simulink model "main"  (R2022a)
settings: Solver=FixedStepDiscrete  StartTime=0.0  StopTime=Inf  FixedStep=(50e-6)-(sim_en*4.995e-5)  RelTol=1e-3  EnableMultiTasking=on
model workspace (MAT data in the model file):
  Param : Simulink.Parameter (value not decoded)
  ac_ok : Simulink.Signal (value not decoded)
  ac_ok_120 : Simulink.Signal (value not decoded)
  bulk_voltage : Simulink.Signal (value not decoded)
  burstduty_integ_max : Simulink.Signal (value not decoded)
  burstduty_integ_min : Simulink.Signal (value not decoded)
  burstduty_ki : Simulink.Signal (value not decoded)
  burstduty_kp : Simulink.Signal (value not decoded)
  calib_ok : Simulink.Signal (value not decoded)
  can_addr1 : Simulink.Signal (value not decoded)
  can_addr2 : Simulink.Signal (value not decoded)
  can_addr3 : Simulink.Signal (value not decoded)
  can_addr4 : Simulink.Signal (value not decoded)
  can_data_rx : Simulink.Signal (value not decoded)
  can_data_tx : Simulink.Signal (value not decoded)
  can_timeout_120 : Simulink.Signal (value not decoded)
  chksum_scircv : Simulink.Signal (value not decoded)
  clllc_en_120 : Simulink.Signal (value not decoded)
  clllc_fault_120 : Simulink.Signal (value not decoded)
  clllc_ok_120 : Simulink.Signal (value not decoded)
  cmpss1h : Simulink.Signal (value not decoded)
  cmpss1l : Simulink.Signal (value not decoded)
  cmpss2h : Simulink.Signal (value not decoded)
  cmpss2l : Simulink.Signal (value not decoded)
  cmpss3h : Simulink.Signal (value not decoded)
  cmpss3l : Simulink.Signal (value not decoded)
  cmpss4h : Simulink.Signal (value not decoded)
  cmpss4l : Simulink.Signal (value not decoded)
  cmpss5h : Simulink.Signal (value not decoded)
  cmpss5l : Simulink.Signal (value not decoded)
  cmpss6h : Simulink.Signal (value not decoded)
  cmpss6l : Simulink.Signal (value not decoded)
  cmpss7h : Simulink.Signal (value not decoded)
  cmpss7l : Simulink.Signal (value not decoded)
  cmpss8h : Simulink.Signal (value not decoded)
  cmpss8l : Simulink.Signal (value not decoded)
  cnt_idle : Simulink.Signal (value not decoded)
  cnt_orps : Simulink.Signal (value not decoded)
  cnt_scircv : Simulink.Signal (value not decoded)
  cnt_scixmt : Simulink.Signal (value not decoded)
  cnt_scixmt_func : Simulink.Signal (value not decoded)
  cnt_temp_mux : Simulink.Signal (value not decoded)
  cnt_vdroop : Simulink.Signal (value not decoded)
  config_ok : Simulink.Signal (value not decoded)
  control_en : Simulink.Signal (value not decoded)
  cp_ready_120 : Simulink.Signal (value not decoded)
  d2d_en : Simulink.Signal (value not decoded)
  dchg_off : Simulink.Signal (value not decoded)
  debug_dacb : Simulink.Signal (value not decoded)
  debug_dacc : Simulink.Signal (value not decoded)
  debug_msg1 : Simulink.Signal (value not decoded)
  debug_msg2 : Simulink.Signal (value not decoded)
  debug_msg3 : Simulink.Signal (value not decoded)
  debug_msg4 : Simulink.Signal (value not decoded)
  debug_msg5 : Simulink.Signal (value not decoded)
  debug_msg6 : Simulink.Signal (value not decoded)
  dir_v2g : Simulink.Signal (value not decoded)
  eoss_llc1 : Simulink.Signal (value not decoded)
  eoss_llc2 : Simulink.Signal (value not decoded)
  eoss_orps : Simulink.Signal (value not decoded)
  fault_ocp : Simulink.Signal (value not decoded)
  fault_otp : Simulink.Signal (value not decoded)
  fault_ovp : Simulink.Signal (value not decoded)
  fut_en : Simulink.Signal (value not decoded)
  fwd_en_120 : Simulink.Signal (value not decoded)
  gain_llc1_sec_idc : Simulink.Signal (value not decoded)
  gain_llc1_temp_sr : Simulink.Signal (value not decoded)
  gain_llc2_sec_idc : Simulink.Signal (value not decoded)
  gain_vbat : Simulink.Signal (value not decoded)
  gain_vbulk : Simulink.Signal (value not decoded)
  gain_vout : Simulink.Signal (value not decoded)
  input_current_phasea : Simulink.Signal (value not decoded)
  input_current_phaseb : Simulink.Signal (value not decoded)
  input_current_phasec : Simulink.Signal (value not decoded)
  input_freq : Simulink.Signal (value not decoded)
  input_power : Simulink.Signal (value not decoded)
  input_voltage_phasea : Simulink.Signal (value not decoded)
  input_voltage_phaseb : Simulink.Signal (value not decoded)
  input_voltage_phasec : Simulink.Signal (value not decoded)
  ishare_arbiter : Simulink.Signal (value not decoded)
  ishare_thresh : Simulink.Signal (value not decoded)
  led_g : Simulink.Signal (value not decoded)
  led_r : Simulink.Signal (value not decoded)
  led_y : Simulink.Signal (value not decoded)
  llc1_burst_integ : Simulink.Signal (value not decoded)
  llc1_burstduty_buffer : Simulink.Signal (value not decoded)
  llc1_pfm_error : Simulink.Signal (value not decoded)
  llc1_pfm_integ : Simulink.Signal (value not decoded)
  llc1_pfm_prop : Simulink.Signal (value not decoded)
  llc1_pri_idc : Simulink.Signal (value not decoded)
  llc1_ps_buffer : Simulink.Signal (value not decoded)
  llc1_pspwm_error : Simulink.Signal (value not decoded)
  llc1_pspwm_integ : Simulink.Signal (value not decoded)
  llc1_pspwm_prop : Simulink.Signal (value not decoded)
  llc1_sec_idc : Simulink.Signal (value not decoded)
  llc1_temp_sr : Simulink.Signal (value not decoded)
  llc1_ts_tbctr_buffer : Simulink.Signal (value not decoded)
  llc2_burst_integ : Simulink.Signal (value not decoded)
  llc2_burstduty_buffer : Simulink.Signal (value not decoded)
  llc2_en : Simulink.Signal (value not decoded)
  llc2_en_buffer : Simulink.Signal (value not decoded)
  llc2_pfm_error : Simulink.Signal (value not decoded)
  llc2_pfm_integ : Simulink.Signal (value not decoded)
  llc2_pfm_prop : Simulink.Signal (value not decoded)
  llc2_pri_idc : Simulink.Signal (value not decoded)
  llc2_ps_buffer : Simulink.Signal (value not decoded)
  llc2_pspwm_error : Simulink.Signal (value not decoded)
  llc2_pspwm_integ : Simulink.Signal (value not decoded)
  llc2_pspwm_prop : Simulink.Signal (value not decoded)
  llc2_sec_idc : Simulink.Signal (value not decoded)
  llc2_temp_sr : Simulink.Signal (value not decoded)
  llc2_ts_tbctr_buffer : Simulink.Signal (value not decoded)
  loop_adcint : Simulink.Signal (value not decoded)
  loop_control : Simulink.Signal (value not decoded)
  loop_idle : Simulink.Signal (value not decoded)
  mid_bulk_voltage : Simulink.Signal (value not decoded)
  mode_120 : Simulink.Signal (value not decoded)
  mode_cc_cv : Simulink.Signal (value not decoded)
  myParam : mpt.Parameter (value not decoded)
  obc_ok_120 : Simulink.Signal (value not decoded)
  offset_llc1_sec_idc : Simulink.Signal (value not decoded)
  offset_llc1_temp_sr : Simulink.Signal (value not decoded)
  offset_llc2_sec_idc : Simulink.Signal (value not decoded)
  offset_vbat : Simulink.Signal (value not decoded)
  offset_vbulk : Simulink.Signal (value not decoded)
  offset_vout : Simulink.Signal (value not decoded)
  openloop_en : Simulink.Signal (value not decoded)
  openloop_fault_en : Simulink.Signal (value not decoded)
  ot_fault_120 : Simulink.Signal (value not decoded)
  pfc_en : Simulink.Signal (value not decoded)
  pfc_en_120 : Simulink.Signal (value not decoded)
  pfc_fw_revision : Simulink.Signal (value not decoded)
  pfc_fw_revision_bootloader : Simulink.Signal (value not decoded)
  pfc_fw_revision_debug : Simulink.Signal (value not decoded)
  pfc_ok : Simulink.Signal (value not decoded)
  pfc_ok_120 : Simulink.Signal (value not decoded)
  pfm_a0 : Simulink.Signal (value not decoded)
  pfm_a1 : Simulink.Signal (value not decoded)
  pfm_integ_max : Simulink.Signal (value not decoded)
  pfm_integ_min : Simulink.Signal (value not decoded)
  pfm_ki : Simulink.Signal (value not decoded)
  pfm_kp : Simulink.Signal (value not decoded)
  pri_fut_en : Simulink.Signal (value not decoded)
  pri_fut_en_buffer : Simulink.Signal (value not decoded)
  pri_halfbridge_en : Simulink.Signal (value not decoded)
  pri_halfbridge_en_buffer : Simulink.Signal (value not decoded)
  pspwm_integ_max : Simulink.Signal (value not decoded)
  pspwm_integ_min : Simulink.Signal (value not decoded)
  pspwm_ki : Simulink.Signal (value not decoded)
  pspwm_kp : Simulink.Signal (value not decoded)
  ref_idclink_max : Simulink.Signal (value not decoded)
  ref_iout : Simulink.Signal (value not decoded)
  ref_iout_calib : Simulink.Signal (value not decoded)
  ref_iout_llc1 : Simulink.Signal (value not decoded)
  ref_iout_llc1_calib : Simulink.Signal (value not decoded)
  ref_iout_llc2 : Simulink.Signal (value not decoded)
  ref_iout_llc2_calib : Simulink.Signal (value not decoded)
  ref_pout : Simulink.Signal (value not decoded)
  ref_ss_llc1 : Simulink.Signal (value not decoded)
  ref_ss_llc2 : Simulink.Signal (value not decoded)
  ref_ss_orps : Simulink.Signal (value not decoded)
  ref_vbat : Simulink.Signal (value not decoded)
  ref_vbat_calib : Simulink.Signal (value not decoded)
  ref_vbulk : Simulink.Signal (value not decoded)
  ref_vbulk_calib : Simulink.Signal (value not decoded)
  ref_vbulk_llc1_calib : Simulink.Signal (value not decoded)
  ref_vbulk_llc2_calib : Simulink.Signal (value not decoded)
  ref_vout : Simulink.Signal (value not decoded)
  ref_vout_calib : Simulink.Signal (value not decoded)
  relay_en : Simulink.Signal (value not decoded)
  reset_flag : Simulink.Signal (value not decoded)
  rev_en_120 : Simulink.Signal (value not decoded)
  runtime_control : Simulink.Signal (value not decoded)
  runtime_idle : Simulink.Signal (value not decoded)
  scircv_buffer : Simulink.Signal (value not decoded)
  scircv_buffer_tmp : Simulink.Signal (value not decoded)
  scircv_buffer_tmp_idx0 : Simulink.Signal (value not decoded)
  scircv_chksum : Simulink.Signal (value not decoded)
  scircv_chksum_ok : Simulink.Signal (value not decoded)
  scircv_parse_ok : Simulink.Signal (value not decoded)
  scixmt_buffer : Simulink.Signal (value not decoded)
  scixmt_chksum : Simulink.Signal (value not decoded)
  scixmt_func : Simulink.Signal (value not decoded)
  scixmt_word0_lsb : Simulink.Signal (value not decoded)
  scixmt_word0_msb : Simulink.Signal (value not decoded)
  scixmt_word1_lsb : Simulink.Signal (value not decoded)
  scixmt_word1_msb : Simulink.Signal (value not decoded)
  scixmt_word2_lsb : Simulink.Signal (value not decoded)
  scixmt_word2_msb : Simulink.Signal (value not decoded)
  scixmt_wr : Simulink.Signal (value not decoded)
  ss_step : Simulink.Signal (value not decoded)
  state_calib : Simulink.Signal (value not decoded)
  state_control : Simulink.Signal (value not decoded)
  state_hkeep : Simulink.Signal (value not decoded)
  status_cmpss : Simulink.Signal (value not decoded)
  status_control : Simulink.Signal (value not decoded)
  status_digin : Simulink.Signal (value not decoded)
  status_digout : Simulink.Signal (value not decoded)
  status_fault : Simulink.Signal (value not decoded)
  status_input : Simulink.Signal (value not decoded)
  status_pfc : Simulink.Signal (value not decoded)
  temp_inlet : Simulink.Signal (value not decoded)
  temp_llc1_fet_hs : Simulink.Signal (value not decoded)
  temp_llc2_fet_hs : Simulink.Signal (value not decoded)
  temp_mux : Simulink.Signal (value not decoded)
  temp_mux_s0 : Simulink.Signal (value not decoded)
  temp_mux_s1 : Simulink.Signal (value not decoded)
  temp_mux_s2 : Simulink.Signal (value not decoded)
  temp_outlet : Simulink.Signal (value not decoded)
  temp_pfc_fet_hsa : Simulink.Signal (value not decoded)
  temp_pfc_fet_hsb : Simulink.Signal (value not decoded)
  temp_pfc_fet_hsc : Simulink.Signal (value not decoded)
  temp_pfc_fet_lsa : Simulink.Signal (value not decoded)
  temp_pfc_fet_lsb : Simulink.Signal (value not decoded)
  temp_pfc_fet_lsc : Simulink.Signal (value not decoded)
  test_mode : Simulink.Signal (value not decoded)
  tfcv_cc : Simulink.Signal (value not decoded)
  tfcv_cc_llc2 : Simulink.Signal (value not decoded)
  tfcv_cv : Simulink.Signal (value not decoded)
  tfcv_sr_en : Simulink.Signal (value not decoded)
  tfv_assert_llc1_pri_idc : Simulink.Signal (value not decoded)
  tfv_assert_llc1_sec_idc : Simulink.Signal (value not decoded)
  tfv_assert_llc1_temp_sr : Simulink.Signal (value not decoded)
  tfv_assert_llc2_pri_idc : Simulink.Signal (value not decoded)
  tfv_assert_llc2_sec_idc : Simulink.Signal (value not decoded)
  tfv_assert_llc2_temp_sr : Simulink.Signal (value not decoded)
  tfv_assert_temp_outlet : Simulink.Signal (value not decoded)
  tfv_assert_vaux_uv : Simulink.Signal (value not decoded)
  tfv_assert_vbat : Simulink.Signal (value not decoded)
  tfv_assert_vbulk : Simulink.Signal (value not decoded)
  tfv_assert_vout : Simulink.Signal (value not decoded)
  tfv_cnt_tz : Simulink.Signal (value not decoded)
  tfv_deassert_llc1_pri_idc : Simulink.Signal (value not decoded)
  tfv_deassert_llc1_sec_idc : Simulink.Signal (value not decoded)
  tfv_deassert_llc1_temp_sr : Simulink.Signal (value not decoded)
  tfv_deassert_llc2_pri_idc : Simulink.Signal (value not decoded)
  tfv_deassert_llc2_sec_idc : Simulink.Signal (value not decoded)
  tfv_deassert_llc2_temp_sr : Simulink.Signal (value not decoded)
  tfv_deassert_temp_outlet : Simulink.Signal (value not decoded)
  tfv_deassert_vaux_uv : Simulink.Signal (value not decoded)
  tfv_deassert_vbat : Simulink.Signal (value not decoded)
  tfv_deassert_vbulk : Simulink.Signal (value not decoded)
  tfv_deassert_vout : Simulink.Signal (value not decoded)
  tfv_llc1_pri_idc : Simulink.Signal (value not decoded)
  tfv_llc1_sec_idc : Simulink.Signal (value not decoded)
  tfv_llc1_temp_sr : Simulink.Signal (value not decoded)
  tfv_llc2_pri_idc : Simulink.Signal (value not decoded)
  tfv_llc2_sec_idc : Simulink.Signal (value not decoded)
  tfv_llc2_temp_sr : Simulink.Signal (value not decoded)
  tfv_temp_outlet : Simulink.Signal (value not decoded)
  tfv_vaux_uv : Simulink.Signal (value not decoded)
  tfv_vbat : Simulink.Signal (value not decoded)
  tfv_vbulk : Simulink.Signal (value not decoded)
  tfv_vout : Simulink.Signal (value not decoded)
  timer_1ms : Simulink.Signal (value not decoded)
  tz : Simulink.Signal (value not decoded)
  valve_en : Simulink.Signal (value not decoded)
  vaux : Simulink.Signal (value not decoded)
  vbat : Simulink.Signal (value not decoded)
  vbulk : Simulink.Signal (value not decoded)
  vout : Simulink.Signal (value not decoded)
undefined symbols (not defined in the file or in its folder): CAN_O_INT, CANA_BASE, Down, GPTRIP1SEL, GPTRIP2SEL, TZ1, TZ2, Up
libraries: hdlsllib x159, simulink x94, c2802xlib x32, c2837xDlib x19, c2807xlib x16, c280xlib x13, canmsglib x8, idelinklib_common x2, c2000lib x1, c281xlib x1
(part 11 of 20)

== system main/Task_Manager/idle/idle_task/hkeep/tz ==
  note: //Code:
      | main_DWork.tz_sc = (uint16_T)(EPwm1Regs.TZOSTFLG.bit.OST1);
      | main_DWork.tz_oc = (uint16_T)(EPwm1Regs.TZOSTFLG.bit.OST2);
      | main_DWork.tz_ov = (uint16_T)(EPwm1Regs.TZOSTFLG.bit.OST3);
  note: main_DWork.tz = (uint16_T)(EPwm1Regs.TZOSTFLG.bit.OST3);
  note: main_DWork.tz = (uint16_T)(EPwm1Regs.TZCBCFLG.bit.CBC3);
  note: //Code:
      | main_DWork.tz_ov = (uint16_T)(EPwm1Regs.TZOSTFLG.bit.OST1); //X-BAR GPIO61 VBULK and VBAT OVP
      | //main_DWork.tz_ocp1 = (uint16_T)(EPwm1Regs.TZOSTFLG.bit.OST2); //X-BAR GPIO62 IOUT OCP
      | //main_DWork.tz_ocp2 = (uint16_T)(EPwm1Regs.TZOSTFLG.bit.OST3); //X-BAR GPIO63 ITANK OCP
  function : TriggerPort  TriggerType=function-call  VariantControl=Variant
  System Outputs : Subsystem  Commented=on  mask(System Outputs){ShowInLibBrowser=0}
      mask prompts: ShowInLibBrowser "Simulink:masks:CustCodeMaskParam1_MP"
      settings: CopyFcn=cccopyfcn(gcb)  OpenFcn=ccopenfcn('System Outputs Function')
      mask Help: eval('feval(''rtwprivate'',''rtwhelpview'',''rtw_sys_outputs_block'')');
      mask Display: disp('System\nOutputs');
  System Outputs1 : Subsystem  Commented=on  mask(System Outputs){ShowInLibBrowser=0}
      mask prompts: ShowInLibBrowser "Simulink:masks:CustCodeMaskParam1_MP"
      settings: CopyFcn=cccopyfcn(gcb)  OpenFcn=ccopenfcn('System Outputs Function')
      mask Help: eval('feval(''rtwprivate'',''rtwhelpview'',''rtw_sys_outputs_block'')');
      mask Display: disp('System\nOutputs');
  System Outputs2 : Subsystem  Commented=on  mask(System Outputs){ShowInLibBrowser=0}
      mask prompts: ShowInLibBrowser "Simulink:masks:CustCodeMaskParam1_MP"
      settings: CopyFcn=cccopyfcn(gcb)  OpenFcn=ccopenfcn('System Outputs Function')
      mask Help: eval('feval(''rtwprivate'',''rtwhelpview'',''rtw_sys_outputs_block'')');
      mask Display: disp('System\nOutputs');
  System Outputs3 : Subsystem  Commented=on  mask(System Outputs){ShowInLibBrowser=0}
      mask prompts: ShowInLibBrowser "Simulink:masks:CustCodeMaskParam1_MP"
      settings: CopyFcn=cccopyfcn(gcb)  OpenFcn=ccopenfcn('System Outputs Function')
      mask Help: eval('feval(''rtwprivate'',''rtwhelpview'',''rtw_sys_outputs_block'')');
      mask Display: disp('System\nOutputs');
  System Outputs4 : Subsystem  mask(System Outputs){ShowInLibBrowser=0}
      mask prompts: ShowInLibBrowser "Simulink:masks:CustCodeMaskParam1_MP"
      settings: CopyFcn=cccopyfcn(gcb)  OpenFcn=ccopenfcn('System Outputs Function')
      mask Help: eval('feval(''rtwprivate'',''rtwhelpview'',''rtw_sys_outputs_block'')');
      mask Display: disp('System\nOutputs');

== system main/Task_Manager/idle/idle_task/status/init ==
  sim_digin : Inport
  function : TriggerPort  TriggerType=function-call  VariantControl=Variant
  digin/digout_variant_subsystem : Subsystem  Variant=on
  sim_digout : Outport
  wires:
  sim_digin/1 -> digin/digout_variant_subsystem/1(sim_digin)
  digin/digout_variant_subsystem/1(sim_digout) -> sim_digout/1

== system main/Task_Manager/idle/idle_task/status/status_control ==
  function : TriggerPort  TriggerType=function-call  VariantControl=Variant
  Add : Sum  Inputs=+++++++++++
  Bit Shift1 : hdlsllib/Logic and Bit Operations/Bit Shift  mode=Shift Left Logical  N=1
  Bit Shift10 : hdlsllib/Logic and Bit Operations/Bit Shift  mode=Shift Left Logical  N=10
  Bit Shift2 : hdlsllib/Logic and Bit Operations/Bit Shift  mode=Shift Left Logical  N=2
  Bit Shift3 : hdlsllib/Logic and Bit Operations/Bit Shift  mode=Shift Left Logical  N=3
  Bit Shift4 : hdlsllib/Logic and Bit Operations/Bit Shift  mode=Shift Left Logical  N=5
  Bit Shift5 : hdlsllib/Logic and Bit Operations/Bit Shift  mode=Shift Left Logical  N=6
  Bit Shift6 : hdlsllib/Logic and Bit Operations/Bit Shift  mode=Shift Left Logical  N=4
  Bit Shift7 : hdlsllib/Logic and Bit Operations/Bit Shift  mode=Shift Left Logical  N=7
  Bit Shift8 : hdlsllib/Logic and Bit Operations/Bit Shift  mode=Shift Left Logical  N=8
  Bit Shift9 : hdlsllib/Logic and Bit Operations/Bit Shift  mode=Shift Left Logical  N=9
  Data Store Read1 : DataStoreRead  DataStoreName=eoss_llc2  IndexOptions=Index vector (dialog)  Indices=1  OutputSizes=1
  Data Store Read10 : DataStoreRead  DataStoreName=dir_v2g  IndexOptions=Index vector (dialog)  Indices=1  OutputSizes=1
  Data Store Read11 : DataStoreRead  DataStoreName=eoss_llc1  IndexOptions=Index vector (dialog)  Indices=1  OutputSizes=1
  Data Store Read12 : DataStoreRead  DataStoreName=calib_ok  IndexOptions=Index vector (dialog)  Indices=1  OutputSizes=1
  Data Store Read13 : DataStoreRead  DataStoreName=openloop_en  IndexOptions=Index vector (dialog)  Indices=1  OutputSizes=1
  Data Store Read2 : DataStoreRead  DataStoreName=llc2_en  IndexOptions=Index vector (dialog)  Indices=1  OutputSizes=1
  Data Store Read3 : DataStoreRead  DataStoreName=pri_halfbridge_en  IndexOptions=Index vector (dialog)  Indices=1  OutputSizes=1
  Data Store Read4 : DataStoreRead  DataStoreName=config_ok  IndexOptions=Index vector (dialog)  Indices=1  OutputSizes=1
  Data Store Read5 : DataStoreRead  DataStoreName=openloop_fault_en  IndexOptions=Index vector (dialog)  Indices=1  OutputSizes=1
  Data Store Read6 : DataStoreRead  DataStoreName=control_en  IndexOptions=Index vector (dialog)  Indices=1  OutputSizes=1
  Data Store Read7 : DataStoreRead  DataStoreName=fut_en  IndexOptions=Index vector (dialog)  Indices=1  OutputSizes=1
  Data Store Write7 : DataStoreWrite  DataStoreName=status_control  IndexOptions=Index vector (dialog)  Indices=1  OutputSizes=1
  Data Type Conversion{,1..10} (11 alike) : DataTypeConversion  OutDataTypeStr=uint16  SaturateOnIntegerOverflow=off  RndMeth=Floor
  wires:
  Add/1 -> Data Store Write7/1
  Data Store Read10/1 -> Data Type Conversion1/1
  Bit Shift2/1 -> Add/3
  Data Store Read6/1 -> Data Type Conversion/1
  Bit Shift3/1 -> Add/4
  Bit Shift1/1 -> Add/2
  Bit Shift6/1 -> Add/5
  Data Type Conversion1/1 -> Bit Shift1/1
  Data Type Conversion2/1 -> Bit Shift2/1
  Data Type Conversion3/1 -> Bit Shift3/1
  Data Type Conversion4/1 -> Bit Shift6/1
  Bit Shift4/1 -> Add/6
  Data Store Read12/1 -> Data Type Conversion2/1
  Data Type Conversion5/1 -> Bit Shift4/1
  Data Type Conversion6/1 -> Bit Shift5/1
  Data Type Conversion7/1 -> Bit Shift7/1
  Data Type Conversion8/1 -> Bit Shift8/1
  Data Type Conversion9/1 -> Bit Shift9/1
  Bit Shift9/1 -> Add/10
  Bit Shift5/1 -> Add/7
  Bit Shift7/1 -> Add/8
  Bit Shift8/1 -> Add/9
  Data Type Conversion/1 -> Add/1
  Data Type Conversion10/1 -> Bit Shift10/1
  Bit Shift10/1 -> Add/11
  Data Store Read3/1 -> Data Type Conversion10/1
  Data Store Read2/1 -> Data Type Conversion9/1
  Data Store Read5/1 -> Data Type Conversion8/1
  Data Store Read13/1 -> Data Type Conversion7/1
  Data Store Read7/1 -> Data Type Conversion6/1
  Data Store Read1/1 -> Data Type Conversion5/1
  Data Store Read11/1 -> Data Type Conversion4/1
  Data Store Read4/1 -> Data Type Conversion3/1

== system main/Task_Manager/idle/idle_task/status/status_digin ==
  function : TriggerPort  TriggerType=function-call  VariantControl=Variant
  Add : Sum  Inputs=+++++++
  Bit Shift1 : hdlsllib/Logic and Bit Operations/Bit Shift  mode=Shift Left Logical  N=1
  Bit Shift2 : hdlsllib/Logic and Bit Operations/Bit Shift  mode=Shift Left Logical  N=2
  Bit Shift3 : hdlsllib/Logic and Bit Operations/Bit Shift  mode=Shift Left Logical  N=3
  Bit Shift4 : hdlsllib/Logic and Bit Operations/Bit Shift  mode=Shift Left Logical  N=5
  Bit Shift5 : hdlsllib/Logic and Bit Operations/Bit Shift  mode=Shift Left Logical  N=6
  Bit Shift6 : hdlsllib/Logic and Bit Operations/Bit Shift  mode=Shift Left Logical  N=4
  Data Store Read : DataStoreRead  DataStoreName=can_addr1  IndexOptions=Index vector (dialog)  Indices=1  OutputSizes=1
  Data Store Read1 : DataStoreRead  DataStoreName=can_addr2  IndexOptions=Index vector (dialog)  Indices=1  OutputSizes=1
  Data Store Read2 : DataStoreRead  DataStoreName=can_addr3  IndexOptions=Index vector (dialog)  Indices=1  OutputSizes=1
  Data Store Read3 : DataStoreRead  DataStoreName=can_addr4  IndexOptions=Index vector (dialog)  Indices=1  OutputSizes=1
  Data Store Read4 : DataStoreRead  DataStoreName=pfc_ok  IndexOptions=Index vector (dialog)  Indices=1  OutputSizes=1
  Data Store Read5 : DataStoreRead  DataStoreName=ac_ok  IndexOptions=Index vector (dialog)  Indices=1  OutputSizes=1
  Data Store Read6 : DataStoreRead  DataStoreName=d2d_en  IndexOptions=Index vector (dialog)  Indices=1  OutputSizes=1
  Data Store Write : DataStoreWrite  DataStoreName=status_digin  IndexOptions=Index vector (dialog)  Indices=1  OutputSizes=1
  Data Type Conversion{,1..6} (7 alike) : DataTypeConversion  OutDataTypeStr=uint16  SaturateOnIntegerOverflow=off  RndMeth=Floor
  wires:
  Data Store Read/1 -> Data Type Conversion/1
  Data Store Read1/1 -> Data Type Conversion1/1
  Data Store Read2/1 -> Data Type Conversion2/1
  Data Store Read6/1 -> Data Type Conversion6/1
  Data Store Read5/1 -> Data Type Conversion5/1
  Data Store Read4/1 -> Data Type Conversion4/1
  Data Store Read3/1 -> Data Type Conversion3/1
  Bit Shift5/1 -> Add/7
  Bit Shift4/1 -> Add/6
  Bit Shift6/1 -> Add/5
  Bit Shift3/1 -> Add/4
  Bit Shift2/1 -> Add/3
  Bit Shift1/1 -> Add/2
  Add/1 -> Data Store Write/1
  Data Type Conversion/1 -> Add/1
  Data Type Conversion1/1 -> Bit Shift1/1
  Data Type Conversion2/1 -> Bit Shift2/1
  Data Type Conversion3/1 -> Bit Shift3/1
  Data Type Conversion4/1 -> Bit Shift6/1
  Data Type Conversion5/1 -> Bit Shift4/1
  Data Type Conversion6/1 -> Bit Shift5/1

== system main/Task_Manager/idle/idle_task/status/status_digout ==
  function : TriggerPort  TriggerType=function-call  VariantControl=Variant
  Add : Sum  Inputs=++++++++++
  Bit Shift1 : hdlsllib/Logic and Bit Operations/Bit Shift  mode=Shift Left Logical  N=1
  Bit Shift2 : hdlsllib/Logic and Bit Operations/Bit Shift  mode=Shift Left Logical  N=2
  Bit Shift3 : hdlsllib/Logic and Bit Operations/Bit Shift  mode=Shift Left Logical  N=3
  Bit Shift4 : hdlsllib/Logic and Bit Operations/Bit Shift  mode=Shift Left Logical  N=5
  Bit Shift5 : hdlsllib/Logic and Bit Operations/Bit Shift  mode=Shift Left Logical  N=6
  Bit Shift6 : hdlsllib/Logic and Bit Operations/Bit Shift  mode=Shift Left Logical  N=4
  Bit Shift7 : hdlsllib/Logic and Bit Operations/Bit Shift  mode=Shift Left Logical  N=7
  Bit Shift8 : hdlsllib/Logic and Bit Operations/Bit Shift  mode=Shift Left Logical  N=8
  Bit Shift9 : hdlsllib/Logic and Bit Operations/Bit Shift  mode=Shift Left Logical  N=9
  Data Store Read1 : DataStoreRead  DataStoreName=relay_en  IndexOptions=Index vector (dialog)  Indices=1  OutputSizes=1
  Data Store Read10 : DataStoreRead  DataStoreName=led_g  IndexOptions=Index vector (dialog)  Indices=1  OutputSizes=1
  Data Store Read11 : DataStoreRead  DataStoreName=led_y  IndexOptions=Index vector (dialog)  Indices=1  OutputSizes=1
  Data Store Read12 : DataStoreRead  DataStoreName=dchg_off  IndexOptions=Index vector (dialog)  Indices=1  OutputSizes=1
  Data Store Read13 : DataStoreRead  DataStoreName=pfc_en  IndexOptions=Index vector (dialog)  Indices=1  OutputSizes=1
  Data Store Read14 : DataStoreRead  DataStoreName=temp_mux_s0  IndexOptions=Index vector (dialog)  Indices=1  OutputSizes=1
  Data Store Read15 : DataStoreRead  DataStoreName=temp_mux_s1  IndexOptions=Index vector (dialog)  Indices=1  OutputSizes=1
  Data Store Read16 : DataStoreRead  DataStoreName=valve_en  IndexOptions=Index vector (dialog)  Indices=1  OutputSizes=1
  Data Store Read17 : DataStoreRead  DataStoreName=temp_mux_s2  IndexOptions=Index vector (dialog)  Indices=1  OutputSizes=1
  Data Store Read6 : DataStoreRead  DataStoreName=led_r  IndexOptions=Index vector (dialog)  Indices=1  OutputSizes=1
  Data Store Write7 : DataStoreWrite  DataStoreName=status_digout  IndexOptions=Index vector (dialog)  Indices=1  OutputSizes=1
  Data Type Conversion{,1..9} (10 alike) : DataTypeConversion  OutDataTypeStr=uint16  SaturateOnIntegerOverflow=off  RndMeth=Floor
  Rate Transition1 : RateTransition  Deterministic=off
  Rate Transition2 : RateTransition  Deterministic=off
  Rate Transition3 : RateTransition  Deterministic=off
  wires:
  Add/1 -> Data Store Write7/1
  Data Store Read11/1 -> Data Type Conversion2/1
  Data Store Read13/1 -> Data Type Conversion4/1
  Data Store Read10/1 -> Data Type Conversion1/1
  Bit Shift2/1 -> Add/3
  Data Store Read6/1 -> Data Type Conversion/1
  Bit Shift5/1 -> Add/7
  Bit Shift4/1 -> Add/6
  Bit Shift3/1 -> Add/4
  Data Store Read14/1 -> Rate Transition1/1
  Bit Shift1/1 -> Add/2
  Data Store Read15/1 -> Rate Transition3/1
  Data Store Read12/1 -> Data Type Conversion3/1
  Bit Shift6/1 -> Add/5
  Data Store Read17/1 -> Rate Transition2/1
  Data Store Read16/1 -> Data Type Conversion8/1
  Bit Shift8/1 -> Add/9
  Bit Shift7/1 -> Add/8
  Data Type Conversion/1 -> Add/1
  Data Type Conversion1/1 -> Bit Shift1/1
  Data Type Conversion2/1 -> Bit Shift2/1
  Data Type Conversion3/1 -> Bit Shift3/1
  Data Type Conversion4/1 -> Bit Shift6/1
  Data Type Conversion5/1 -> Bit Shift4/1
  Data Type Conversion6/1 -> Bit Shift5/1
  Data Type Conversion7/1 -> Bit Shift7/1
  Data Type Conversion8/1 -> Bit Shift8/1
  Data Store Read1/1 -> Data Type Conversion9/1
  Bit Shift9/1 -> Add/10
  Data Type Conversion9/1 -> Bit Shift9/1
  Rate Transition1/1 -> Data Type Conversion5/1
  Rate Transition3/1 -> Data Type Conversion6/1
  Rate Transition2/1 -> Data Type Conversion7/1

== system main/Task_Manager/idle/idle_task/status/status_fault ==
  function : TriggerPort  TriggerType=function-call  VariantControl=Variant
  Add1 : Sum  Inputs=++++++++++++
  Bit Shift15 : hdlsllib/Logic and Bit Operations/Bit Shift  mode=Shift Left Logical  N=1
  Bit Shift16 : hdlsllib/Logic and Bit Operations/Bit Shift  mode=Shift Left Logical  N=9
  Bit Shift17 : hdlsllib/Logic and Bit Operations/Bit Shift  mode=Shift Left Logical  N=10
  Bit Shift18 : hdlsllib/Logic and Bit Operations/Bit Shift  mode=Shift Left Logical  N=11
  Bit Shift21 : hdlsllib/Logic and Bit Operations/Bit Shift  mode=Shift Left Logical  N=2
  Bit Shift22 : hdlsllib/Logic and Bit Operations/Bit Shift  mode=Shift Left Logical  N=3
  Bit Shift23 : hdlsllib/Logic and Bit Operations/Bit Shift  mode=Shift Left Logical  N=5
  Bit Shift24 : hdlsllib/Logic and Bit Operations/Bit Shift  mode=Shift Left Logical  N=6
  Bit Shift25 : hdlsllib/Logic and Bit Operations/Bit Shift  mode=Shift Left Logical  N=4
  Bit Shift27 : hdlsllib/Logic and Bit Operations/Bit Shift  mode=Shift Left Logical  N=7
  Bit Shift28 : hdlsllib/Logic and Bit Operations/Bit Shift  mode=Shift Left Logical  N=8
  Data Store Read1 : DataStoreRead  DataStoreName=tfv_llc2_pri_idc  IndexOptions=Index vector (dialog)  Indices=1  OutputSizes=1
  Data Store Read16 : DataStoreRead  DataStoreName=tfv_llc1_sec_idc  IndexOptions=Index vector (dialog)  Indices=1  OutputSizes=1
  Data Store Read17 : DataStoreRead  DataStoreName=tfv_temp_outlet  IndexOptions=Index vector (dialog)  Indices=1  OutputSizes=1
  Data Store Read18 : DataStoreRead  DataStoreName=tfv_llc1_pri_idc  IndexOptions=Index vector (dialog)  Indices=1  OutputSizes=1
  Data Store Read19 : DataStoreRead  DataStoreName=tfv_llc1_temp_sr  IndexOptions=Index vector (dialog)  Indices=1  OutputSizes=1
  Data Store Read20 : DataStoreRead  DataStoreName=tfv_llc2_sec_idc  IndexOptions=Index vector (dialog)  Indices=1  OutputSizes=1
  Data Store Read22 : DataStoreRead  DataStoreName=tfv_vbat  IndexOptions=Index vector (dialog)  Indices=1  OutputSizes=1
  Data Store Read23 : DataStoreRead  DataStoreName=tfv_vout  IndexOptions=Index vector (dialog)  Indices=1  OutputSizes=1
  Data Store Read24 : DataStoreRead  DataStoreName=tfv_llc2_temp_sr  IndexOptions=Index vector (dialog)  Indices=1  OutputSizes=1
  Data Store Read25 : DataStoreRead  DataStoreName=tfv_vbulk  IndexOptions=Index vector (dialog)  Indices=1  OutputSizes=1
  Data Store Read27 : DataStoreRead  DataStoreName=tz  IndexOptions=Index vector (dialog)  Indices=1  OutputSizes=1
  Data Store Read29 : DataStoreRead  DataStoreName=tfv_vaux_uv  IndexOptions=Index vector (dialog)  Indices=1  OutputSizes=1
  Data Store Write1 : DataStoreWrite  DataStoreName=status_fault  IndexOptions=Index vector (dialog)  Indices=1  OutputSizes=1
  Data Type Conversion{15..18,22..29} (12 alike) : DataTypeConversion  OutDataTypeStr=uint16  SaturateOnIntegerOverflow=off  RndMeth=Floor
  wires:
  Data Store Read23/1 -> Data Type Conversion16/1
  Bit Shift17/1 -> Add1/11
  Data Type Conversion17/1 -> Bit Shift17/1
  Data Store Read16/1 -> Data Type Conversion25/1
  Data Type Conversion22/1 -> Bit Shift21/1
  Bit Shift16/1 -> Add1/10
  Bit Shift28/1 -> Add1/9
  Data Store Read18/1 -> Data Type Conversion27/1
  Data Type Conversion24/1 -> Bit Shift25/1
  Data Store Read17/1 -> Data Type Conversion18/1
  Bit Shift22/1 -> Add1/4
  Data Store Read29/1 -> Data Type Conversion24/1
  Data Type Conversion25/1 -> Bit Shift23/1
  Data Type Conversion23/1 -> Bit Shift22/1
  Data Store Read1/1 -> Data Type Conversion28/1
  Data Store Read24/1 -> Data Type Conversion17/1
  Data Store Read19/1 -> Data Type Conversion29/1
  Bit Shift24/1 -> Add1/7
  Data Type Conversion16/1 -> Bit Shift15/1
  Bit Shift25/1 -> Add1/5
  Data Type Conversion27/1 -> Bit Shift27/1
  Bit Shift21/1 -> Add1/3
  Bit Shift27/1 -> Add1/8
  Data Type Conversion18/1 -> Bit Shift18/1
  Data Type Conversion28/1 -> Bit Shift28/1
  Bit Shift18/1 -> Add1/12
  Data Store Read22/1 -> Data Type Conversion22/1
  Bit Shift23/1 -> Add1/6
  Data Type Conversion26/1 -> Bit Shift24/1
  Data Type Conversion15/1 -> Add1/1
  Data Type Conversion29/1 -> Bit Shift16/1
  Bit Shift15/1 -> Add1/2
  Data Store Read20/1 -> Data Type Conversion26/1
  Data Store Read25/1 -> Data Type Conversion23/1
  Data Store Read27/1 -> Data Type Conversion15/1
  Add1/1 -> Data Store Write1/1

== system main/Task_Manager/idle/idle_task/status/update_CAN_msg1 ==
  note: Boot. Image
  note: MCU ID:-
  note: App. Image
  note: " 1.2.a"
  note: For MSG ID 0x144
  note: Update FW Revision
  note: Project ID:-
  note: (1-PRI., 2-SEC., 3-APM
  note: (1-11kW, 2-22kW)
  note: " 1.0.a"
  note: Revision History:
      | .
      | 1.1c - 3/1/23>11:36am - For A2 Iout Gain & Offset Updated
      | CV mode Disabled
      | 1.1c - 3/1/23>12:19pm - Burst Clamp Removed
      | 1.1d - 3/1/23>10:08pm - SR Disable Logic Updated in Burst
      | Added Integral to Burst CL
      | Temp: BUrst Mode Clmaped
      | Burst Duty Clamped in PC - 60
      | Burst Duty Clamped in CL - 90
      | 1.1e - 4/1/23>10:26pm - +1.1d => Added SS with Delay for Smooth
      | SS and SS Step added from Ref instead of FB.
      | (For Testing) - Test Ok
      |
      | 1.1f - 6/1/23>15:47pm - +1.1e => Fixed PS Config. +
      | OL test Mode also updated with other multiple udates.
      | 1.1g - 9/1/23> 3.02pm - +1.1f => All Enabled with Default DI Signal.
      |
      | 1.1h - 9/1/23> 3.47 pm - +1.1g => All Enabled with DIO Signal enabled too for integration test.
      | 1.1i - 10/1/23> 1.15 am - +1.1g => All Enabled with Integral input for PS and PFM Control Routine
      |
      | 1.2a -10/1/23> am - +.1g => All Enabled with Integral Input for PS and PFM Control Routine and DI Signals Enabled for
      | Integration.
  function : TriggerPort  TriggerType=function-call  VariantControl=Variant
  Constant : Constant  Value=[0x31 0x30 0x61 ]  OutDataTypeStr=uint8  SampleTime=-1
  Constant32 : Constant  Value=[0x31 0x32 0x61]  OutDataTypeStr=uint8  SampleTime=-1
  Constant33 : Constant  Value=[0x31]  OutDataTypeStr=uint8  SampleTime=-1
  Constant34 : Constant  Value=[0x32 ]  OutDataTypeStr=uint8  SampleTime=-1
  Data Store Write31 : DataStoreWrite  DataStoreName=u8FwRevData  IndexOptions=Index vector (dialog)  Indices=1  OutputSizes=1
  OBC_CTRL_MSG_100 : Subsystem  TreatAsAtomicUnit=on
      settings: RTWSystemCode=Inline
  OBC_SEC_DATA1_140 : Subsystem  TreatAsAtomicUnit=on
      settings: RTWSystemCode=Inline
  OBC_SEC_DATA2_141 : Subsystem  TreatAsAtomicUnit=on
      settings: RTWSystemCode=Inline
  OBC_SEC_DATA3_142 : Subsystem  TreatAsAtomicUnit=on
      settings: RTWSystemCode=Inline
  OBC_SEC_DATA4_143 : Subsystem  TreatAsAtomicUnit=on
      settings: RTWSystemCode=Inline
  OBC_SEC_REQ_DEBUG_DATA_146_147 : Subsystem  TreatAsAtomicUnit=on
      settings: RTWSystemCode=Inline
  OBC_SEC_STAT_MSG_120 : Subsystem  TreatAsAtomicUnit=on
      settings: RTWSystemCode=Inline
  Vector Concatenate : Concatenate  NumInputs=4
  wires:
  Vector Concatenate/1 -> Data Store Write31/1
  Constant34/1 -> Vector Concatenate/3
  Constant32/1 -> Vector Concatenate/4
  Constant/1 -> Vector Concatenate/1
  Constant33/1 -> Vector Concatenate/2

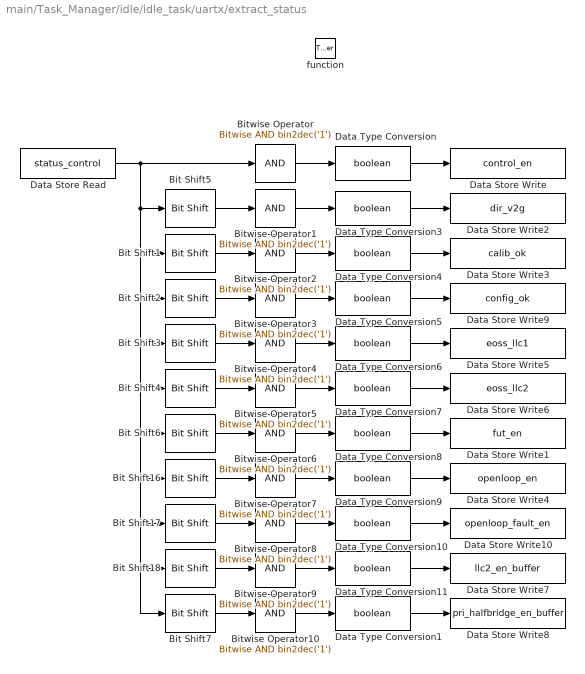
== system main/Task_Manager/idle/idle_task/uartx/extract_status ==
  function : TriggerPort  TriggerType=function-call  VariantControl=Variant
  Bit Shift1 : hdlsllib/Logic and Bit Operations/Bit Shift  mode=Shift Right Logical  N=2
  Bit Shift16 : hdlsllib/Logic and Bit Operations/Bit Shift  mode=Shift Right Logical  N=7
  Bit Shift17 : hdlsllib/Logic and Bit Operations/Bit Shift  mode=Shift Right Logical  N=8
  Bit Shift18 : hdlsllib/Logic and Bit Operations/Bit Shift  mode=Shift Right Logical  N=9
  Bit Shift2 : hdlsllib/Logic and Bit Operations/Bit Shift  mode=Shift Right Logical  N=3
  Bit Shift3 : hdlsllib/Logic and Bit Operations/Bit Shift  mode=Shift Right Logical  N=4
  Bit Shift4 : hdlsllib/Logic and Bit Operations/Bit Shift  mode=Shift Right Logical  N=5
  Bit Shift5 : hdlsllib/Logic and Bit Operations/Bit Shift  mode=Shift Right Logical  N=1
  Bit Shift6 : hdlsllib/Logic and Bit Operations/Bit Shift  mode=Shift Right Logical  N=6
  Bit Shift7 : hdlsllib/Logic and Bit Operations/Bit Shift  mode=Shift Right Logical  N=10
  Bitwise Operator{,1..10} (11 alike) : simulink/Logic and Bit Operations/Bitwise Operator  logicop=AND  UseBitMask=on  BitMask=bin2dec('1')  BitMaskRealWorld=Stored Integer
  Data Store Read : DataStoreRead  DataStoreName=status_control  IndexOptions=Index vector (dialog)  Indices=1  OutputSizes=1
  Data Store Write : DataStoreWrite  DataStoreName=control_en  IndexOptions=Index vector (dialog)  Indices=1  OutputSizes=1
  Data Store Write1 : DataStoreWrite  DataStoreName=fut_en  IndexOptions=Index vector (dialog)  Indices=1  OutputSizes=1
  Data Store Write10 : DataStoreWrite  DataStoreName=openloop_fault_en  IndexOptions=Index vector (dialog)  Indices=1  OutputSizes=1
  Data Store Write2 : DataStoreWrite  DataStoreName=dir_v2g  IndexOptions=Index vector (dialog)  Indices=1  OutputSizes=1
  Data Store Write3 : DataStoreWrite  DataStoreName=calib_ok  IndexOptions=Index vector (dialog)  Indices=1  OutputSizes=1
  Data Store Write4 : DataStoreWrite  DataStoreName=openloop_en  IndexOptions=Index vector (dialog)  Indices=1  OutputSizes=1
  Data Store Write5 : DataStoreWrite  DataStoreName=eoss_llc1  IndexOptions=Index vector (dialog)  Indices=1  OutputSizes=1
  Data Store Write6 : DataStoreWrite  DataStoreName=eoss_llc2  IndexOptions=Index vector (dialog)  Indices=1  OutputSizes=1
  Data Store Write7 : DataStoreWrite  DataStoreName=llc2_en_buffer  IndexOptions=Index vector (dialog)  Indices=1  OutputSizes=1
  Data Store Write8 : DataStoreWrite  DataStoreName=pri_halfbridge_en_buffer  IndexOptions=Index vector (dialog)  Indices=1  OutputSizes=1
  Data Store Write9 : DataStoreWrite  DataStoreName=config_ok  IndexOptions=Index vector (dialog)  Indices=1  OutputSizes=1
  Data Type Conversion{,1,3..11} (11 alike) : DataTypeConversion  OutDataTypeStr=boolean  SaturateOnIntegerOverflow=off  RndMeth=Floor
  wires:
  Bitwise Operator/1 -> Data Type Conversion/1
  Bit Shift5/1 -> Bitwise Operator1/1
  Bit Shift1/1 -> Bitwise Operator2/1
  Bit Shift2/1 -> Bitwise Operator3/1
  Bit Shift3/1 -> Bitwise Operator4/1
  Bit Shift4/1 -> Bitwise Operator5/1
  Bit Shift6/1 -> Bitwise Operator6/1
  Bit Shift16/1 -> Bitwise Operator7/1
  Bit Shift17/1 -> Bitwise Operator8/1
  Bit Shift18/1 -> Bitwise Operator9/1
  Bitwise Operator1/1 -> Data Type Conversion3/1
  Bitwise Operator2/1 -> Data Type Conversion4/1
  Bitwise Operator3/1 -> Data Type Conversion5/1
  Data Type Conversion3/1 -> Data Store Write2/1
  Data Type Conversion4/1 -> Data Store Write3/1
  Bitwise Operator4/1 -> Data Type Conversion6/1
  Bitwise Operator5/1 -> Data Type Conversion7/1
  Bitwise Operator6/1 -> Data Type Conversion8/1
  Bitwise Operator7/1 -> Data Type Conversion9/1
  Bitwise Operator8/1 -> Data Type Conversion10/1
  Bitwise Operator9/1 -> Data Type Conversion11/1
  Bitwise Operator10/1 -> Data Type Conversion1/1
  Data Store Read/1 -> Bit Shift17/1, Bit Shift7/1, Bit Shift18/1, Bit Shift16/1, Bit Shift6/1, Bit Shift4/1, Bit Shift3/1, Bit Shift2/1, Bit Shift1/1, Bit Shift5/1, Bitwise Operator/1
  Bit Shift7/1 -> Bitwise Operator10/1
  Data Type Conversion/1 -> Data Store Write/1
  Data Type Conversion5/1 -> Data Store Write9/1
  Data Type Conversion6/1 -> Data Store Write5/1
  Data Type Conversion7/1 -> Data Store Write6/1
  Data Type Conversion8/1 -> Data Store Write1/1
  Data Type Conversion9/1 -> Data Store Write4/1
  Data Type Conversion10/1 -> Data Store Write10/1
  Data Type Conversion11/1 -> Data Store Write7/1
  Data Type Conversion1/1 -> Data Store Write8/1

== system main/Task_Manager/idle/idle_task/uartx/parse ==
  function : TriggerPort  TriggerType=function-call  VariantControl=Variant
  System Outputs3 : Subsystem  mask(System Outputs){ShowInLibBrowser=0}
      mask prompts: ShowInLibBrowser "Simulink:masks:CustCodeMaskParam1_MP"
      settings: CopyFcn=cccopyfcn(gcb)  OpenFcn=ccopenfcn('System Outputs Function')
      mask Help: eval('feval(''rtwprivate'',''rtwhelpview'',''rtw_sys_outputs_block'')');
      mask Display: disp('System\nOutputs');

== system main/Task_Manager/idle/idle_task/uartx/uart_xmt ==
  function : TriggerPort  TriggerType=function-call  VariantControl=Variant

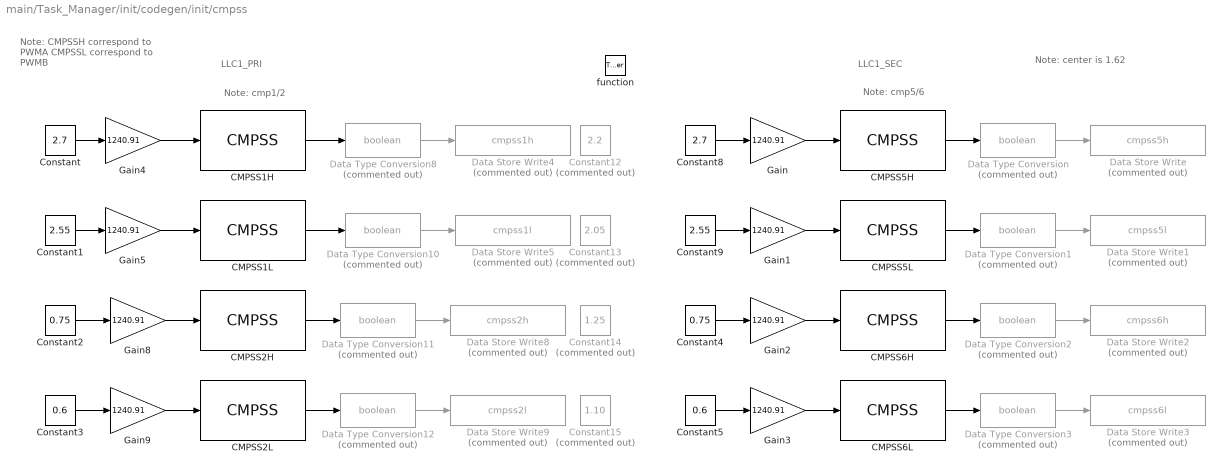
== system main/Task_Manager/init/codegen/init/cmpss ==
  note: Note:
      | center is 1.62
  note: Note:
      | CMPSSH correspond to PWMA
      | CMPSSL correspond to PWMB
  note: LLC1_PRI
  note: LLC1_SEC
  note: Note: cmp1/2
  note: Note: cmp5/6
  function : TriggerPort  TriggerType=function-call  VariantControl=Variant
  CMPSS1H : c2837xDlib/CMPSS  Module=CMPSS1_COMPH  NegativeInput=Internal DAC  DacValueSourceSel=DAC module  DacValueVia=Input port  DACHValue=2234  DACLValue=0  RampMaxRefVal=0  RampDecVal=0  RampDelayVal=0  EnableLatchOut=off  EnableLatchClear=off  SampleTime=-1
      settings: SourceProductBaseCode=TIC2000
  CMPSS1L : c2837xDlib/CMPSS  Module=CMPSS1_COMPL  NegativeInput=Internal DAC  DacValueSourceSel=DAC module  DacValueVia=Input port  DACHValue=2234  DACLValue=0  RampMaxRefVal=0  RampDecVal=0  RampDelayVal=0  EnableLatchOut=off  EnableLatchClear=off  SampleTime=-1
      settings: SourceProductBaseCode=TIC2000
  CMPSS2H : c2837xDlib/CMPSS  Module=CMPSS2_COMPH  NegativeInput=Internal DAC  DacValueSourceSel=DAC module  DacValueVia=Input port  DACHValue=2234  DACLValue=0  RampMaxRefVal=0  RampDecVal=0  RampDelayVal=0  EnableLatchOut=off  EnableLatchClear=off  SampleTime=-1
      settings: SourceProductBaseCode=TIC2000
  CMPSS2L : c2837xDlib/CMPSS  Module=CMPSS2_COMPL  NegativeInput=Internal DAC  DacValueSourceSel=DAC module  DacValueVia=Input port  DACHValue=2234  DACLValue=0  RampMaxRefVal=0  RampDecVal=0  RampDelayVal=0  EnableLatchOut=off  EnableLatchClear=off  SampleTime=-1
      settings: SourceProductBaseCode=TIC2000
  CMPSS5H : c2837xDlib/CMPSS  Module=CMPSS5_COMPH  NegativeInput=Internal DAC  DacValueSourceSel=DAC module  DacValueVia=Input port  DACHValue=2234  DACLValue=0  RampMaxRefVal=0  RampDecVal=0  RampDelayVal=0  EnableLatchOut=off  EnableLatchClear=off  SampleTime=-1
      settings: SourceProductBaseCode=TIC2000
  CMPSS5L : c2837xDlib/CMPSS  Module=CMPSS5_COMPL  NegativeInput=Internal DAC  DacValueSourceSel=DAC module  DacValueVia=Input port  DACHValue=2234  DACLValue=0  RampMaxRefVal=0  RampDecVal=0  RampDelayVal=0  EnableLatchOut=off  EnableLatchClear=off  SampleTime=-1
      settings: SourceProductBaseCode=TIC2000
  CMPSS6H : c2837xDlib/CMPSS  Module=CMPSS6_COMPH  NegativeInput=Internal DAC  DacValueSourceSel=DAC module  DacValueVia=Input port  DACHValue=2234  DACLValue=0  RampMaxRefVal=0  RampDecVal=0  RampDelayVal=0  EnableLatchOut=off  EnableLatchClear=off  SampleTime=-1
      settings: SourceProductBaseCode=TIC2000
  CMPSS6L : c2837xDlib/CMPSS  Module=CMPSS6_COMPL  NegativeInput=Internal DAC  DacValueSourceSel=DAC module  DacValueVia=Input port  DACHValue=2234  DACLValue=0  RampMaxRefVal=0  RampDecVal=0  RampDelayVal=0  EnableLatchOut=off  EnableLatchClear=off  SampleTime=-1
      settings: SourceProductBaseCode=TIC2000
  Constant : Constant  Value=2.7
  Constant1 : Constant  Value=2.55
  Constant12 : Constant  Commented=on  Value=2.2
  Constant13 : Constant  Commented=on  Value=2.05
  Constant14 : Constant  Commented=on  Value=1.25
  Constant15 : Constant  Commented=on  Value=1.10
  Constant2 : Constant  Value=0.75
  Constant3 : Constant  Value=0.6
  Constant4 : Constant  Value=0.75
  Constant5 : Constant  Value=0.6
  Constant8 : Constant  Value=2.7
  Constant9 : Constant  Value=2.55
  Data Store Write : DataStoreWrite  Commented=on  DataStoreName=cmpss5h  IndexOptions=Index vector (dialog)  Indices=1  OutputSizes=1
  Data Store Write1 : DataStoreWrite  Commented=on  DataStoreName=cmpss5l  IndexOptions=Index vector (dialog)  Indices=1  OutputSizes=1
  Data Store Write2 : DataStoreWrite  Commented=on  DataStoreName=cmpss6h  IndexOptions=Index vector (dialog)  Indices=1  OutputSizes=1
  Data Store Write3 : DataStoreWrite  Commented=on  DataStoreName=cmpss6l  IndexOptions=Index vector (dialog)  Indices=1  OutputSizes=1
  Data Store Write4 : DataStoreWrite  Commented=on  DataStoreName=cmpss1h  IndexOptions=Index vector (dialog)  Indices=1  OutputSizes=1
  Data Store Write5 : DataStoreWrite  Commented=on  DataStoreName=cmpss1l  IndexOptions=Index vector (dialog)  Indices=1  OutputSizes=1
  Data Store Write8 : DataStoreWrite  Commented=on  DataStoreName=cmpss2h  IndexOptions=Index vector (dialog)  Indices=1  OutputSizes=1
  Data Store Write9 : DataStoreWrite  Commented=on  DataStoreName=cmpss2l  IndexOptions=Index vector (dialog)  Indices=1  OutputSizes=1
  Data Type Conversion{,1..3,8,10..12} (8 alike) : DataTypeConversion  Commented=on  OutDataTypeStr=boolean  SaturateOnIntegerOverflow=off  RndMeth=Floor
  Gain{,1..5,8..9} (8 alike) : Gain  Gain=1240.91
  wires:
  Constant/1 -> Gain4/1
  Constant1/1 -> Gain5/1
  Gain/1 -> CMPSS5H/1
  Gain1/1 -> CMPSS5L/1
  Gain2/1 -> CMPSS6H/1
  Gain3/1 -> CMPSS6L/1
  CMPSS5H/1 -> Data Type Conversion/1
  CMPSS5L/1 -> Data Type Conversion1/1
  CMPSS6H/1 -> Data Type Conversion2/1
  CMPSS6L/1 -> Data Type Conversion3/1
  CMPSS1H/1 -> Data Type Conversion8/1
  CMPSS1L/1 -> Data Type Conversion10/1
  Gain4/1 -> CMPSS1H/1
  Gain5/1 -> CMPSS1L/1
  CMPSS2L/1 -> Data Type Conversion12/1
  CMPSS2H/1 -> Data Type Conversion11/1
  Gain9/1 -> CMPSS2L/1
  Gain8/1 -> CMPSS2H/1
  Constant3/1 -> Gain9/1
  Constant2/1 -> Gain8/1
  Data Type Conversion/1 -> Data Store Write/1
  Data Type Conversion1/1 -> Data Store Write1/1
  Data Type Conversion3/1 -> Data Store Write3/1
  Data Type Conversion2/1 -> Data Store Write2/1
  Data Type Conversion8/1 -> Data Store Write4/1
  Data Type Conversion10/1 -> Data Store Write5/1
  Data Type Conversion11/1 -> Data Store Write8/1
  Data Type Conversion12/1 -> Data Store Write9/1
  Constant4/1 -> Gain2/1
  Constant5/1 -> Gain3/1
  Constant9/1 -> Gain1/1
  Constant8/1 -> Gain/1
